simulink library "LibraryExperimental"  (R2013b)
settings: Solver=ode45  StartTime=0.0  StopTime=10.0  RelTol=1e-3
values from neighbouring files (symbols this model uses):
  dimActuator = 24    [init_experimental_setup.m]
  layoutActuator = actuatorPlace    [init_experimental_setup.m]
undefined symbols (not defined in the file or in its folder): ident_normalized_static, ultidyn
undefined symbols (not defined in the file): delayWavefrontEthernet, dimSlopeMatrix, dimSquareMatrix, DMmodel, DMmodel_static, sampleTimeTipTilt, sampleTimeWavefrontSensor, staticDMInput, strokeTipTiltMirror
libraries: RCTblocks x1
settings Model: Creator=smauch  LastModifiedBy=smauch

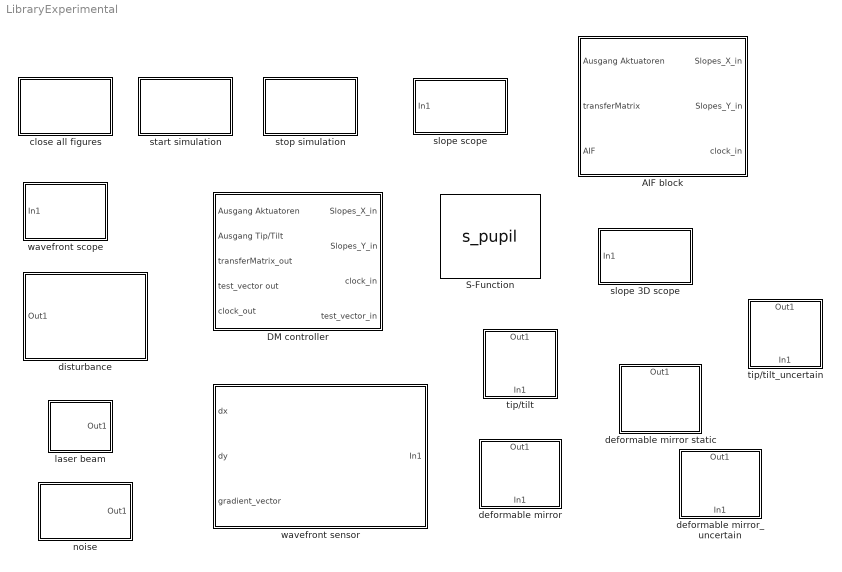
== system LibraryExperimental ==
  AIF block : Subsystem  mask{nbAct=24}
      mask prompts: nbAct "number of actuators"
      mask Display:
      | image(imread('controller.jpg'))
      | color('blue');
      | patch( [0 0.3 0.3 0], [0.9 0.9 0.75 0.75], [0.9, 0.9, 0.9] )
      | port_label('output', 1, 'y')
      | patch( [0 0.5 0.5 0], [0.425 0.425 0.575 0.575], [0.9, 0.9, 0.9] )
      | port_label('output', 2, 'actuator_matrix')
      | patch( [0 0.5 0.5 0], [0.1 0.1 0.25 0.25], [0.9, 0.9, 0.9] )
      | port_label('output', 3, 'AIF_matrix')
      | 
      | patch( [1 0.875 0.875 1], [0.9 0.9 0.75 0.75], [0.9, 0.9, 0.9] )
      | port_label('input', 1, 'dx')
      | patch( [1 0.875 0.875 1], [0.45 0.45 0.55 0.55], [0.9, 0.9, 0.9] )
      | port_label('input', 2, 'dy')
      | patch( [1 0.8 0.8 1], [0.1 0.1 0.25 0.25], [0.9, 0.9, 0.9] )
      | port_label('input', 3, 'clock')
  DM controller : Subsystem
      mask Display:
      | image(imread('controller.jpg'))
      | color('blue');
      | port_label('output', 1, 'y')
      | port_label('output', 2, 'tip/tilt')
      | port_label('output', 3, 'actuator_matrix')
      | 
      | port_label('input', 1, 'dx')
      | port_label('input', 2, 'dy')
      | port_label('input', 3, 'clock')
  S-Function : S-Function  FunctionName=s_pupil  Parameters=dimMatrix  EnableBusSupport=off  mask{dimMatrix=dimSquareMatrix}
      mask prompts: dimMatrix "dimension of input/outut matrix"
      mask Display:
      | t = 0:0.1:2*pi;
      | x = (cos(t)+1)/2;
      | y = (sin(t)+1)/2;
      | patch(x,y,[0 0 0])
      | color('white')
      | fprintf('round\npupil')
  close all figures : Subsystem
      settings: OpenFcn=close all;
      mask Display:
      | patch([0 0 1 1], [0 20 20 0],[1 0 0])
      | color('black')
      | fprintf('close all\nfigures')
  deformable mirror : Subsystem  mask{dimActuator=dimActuator, dimMatrix=dimSquareMatrix, layoutActuator=layoutActuator, model=DMmodel}
      mask prompts: dimActuator "# Actuator"; dimMatrix "dimSquareMatrix"; layoutActuator "layout actuator to dimSquareMatrix"; model "state space model"
      mask Display:
      | image(imread('dm.jpg'))
      | color('white');
      | 
      | port_label('output', 1, 'y')
      | port_label('input', 1, 'u')
      | 
      | patch( [0.15 0.85 0.85 0.15], [0.2 0.2 0.8 0.8], [0 0 0])
      | color('white');
      | fprintf('level 2\ns-function\nuncertain')
  deformable mirror static : Subsystem  mask{dimActuator=dimActuator, dimMatrix=dimSquareMatrix, layoutActuator=layoutActuator, dm_static=DMmodel_static, input=staticDMInput, delay=1}
      mask prompts: dimActuator "# Actuator"; dimMatrix "dimSquareMatrix"; layoutActuator "layout actuator to dimSquareMatrix"; dm_static "static DM model"; input "input for static DM"; delay "delay of disturbance in seconds"
      mask Display:
      | image(imread('dm.jpg'))
      | color('white');
      | 
      | port_label('output', 1, 'y')
      | 
      | patch( [0.15 0.85 0.85 0.15], [0.2 0.2 0.8 0.8], [0 0 0])
      | color('white');
      | fprintf('level 2\ns-function\nstatic')
  deformable mirror_uncertain : Subsystem  AncestorBlock=LibraryExperimental/deformable mirror  mask{Parameter6=0, dimMatrix=dimSquareMatrix, layoutActuator=layoutActuator, model=DMmodel, uncertainty=1/5, ident_normalized_static=ident_normalized_static}
      mask prompts: dimMatrix "dimSquareMatrix"; layoutActuator "layout actuator to dimSquareMatrix"; model "state space model"; uncertainty "uncertainty (normalized)"
      mask Display:
      | image(imread('dm.jpg'))
      | color('white');
      | 
      | port_label('output', 1, 'y')
      | port_label('input', 1, 'u')
      | 
      | patch( [0.15 0.85 0.85 0.15], [0.2 0.2 0.8 0.8], [0 0 0])
      | color('white');
      | fprintf('level 2\ns-function\nuncertain')
  disturbance : Subsystem  mask{dimMatrix=dimSquareMatrix, zernik1=1, zernik2=-1, scale=5, rotate=45}
      mask prompts: dimMatrix "dimSquareMatrix"; zernik1 "Zernike1"; zernik2 "Zernike2"; rotate "rotate in deg"
      mask Display:
      | port_label('output', 1, 'y')
      | 
      | patch([0 0.5 1], [0 1 0],[0.7 0.6 0])
      | patch( [0.15 0.85 0.85 0.15], [0.6 0.6 0.4 0.4], [0.9 0.9 0.9] )
      | fprintf('stationar Zernike')
  laser beam : Subsystem  mask{dimSquare=dimSquareMatrix}
      mask prompts: dimSquare "dimSquareMatrix"
      mask Display:
      | %patch([0 0.5 1], [0 1 0],[0.9 0.3 0.5])
      | image('laser.jpg')
      | patch( [0 1 1 0], [0.8 0.8 0.45 0.45], [0.9 0.9 0.9] )
      | fprintf('laser beam\n')
  noise : Subsystem  mask{enable=on, dimSquare=dimSquareMatrix, Ts=-1, scaleNoise=1}
      mask prompts: enable "enable noise"; dimSquare "dimSquareMatrix"; Ts "sample time"; scaleNoise "noise scaling (default is rand)"
      mask Display:
      | patch([0 0.5 1], [0 1 0],[0.9 0.3 0.5])
      | patch( [0.15 0.85 0.85 0.15], [0.75 0.75 0.25 0.25], [0.9 0.9 0.9] )
      | fprintf('noise\ngeneration')
  slope 3D scope : Subsystem  mask{sampleTime=0.1, dimMatrix=dimSlopeMatrix, enable=on, title='3D wavefront sensor'}
      mask prompts: sampleTime "Sample Time"; dimMatrix "dimSquareMatrix"; enable "enable Scope"
      mask Display:
      | patch([0 0.5 1], [0 1 0],[1 0 0])
      | patch( [0.15 0.85 0.85 0.15], [0.6 0.6 0.4 0.4], [0.9 0.9 0.9] )
      | fprintf('Scope 3D SHWFS')
  slope scope : Subsystem  mask{sampleTime=0.1, dimMatrix=dimSlopeMatrix, enable=on, title='wavefront sensor'}
      mask prompts: sampleTime "Sample Time"; dimMatrix "dimSquareMatrix"; enable "enable Scope"
      mask Display:
      | patch([0 0.5 1], [0 1 0],[1 0 0])
      | patch( [0.15 0.85 0.85 0.15], [0.6 0.6 0.4 0.4], [0.9 0.9 0.9] )
      | fprintf('Scope Quiver')
  start simulation : Subsystem
      settings: OpenFcn=set_param(gcs, 'SimulationCommand', 'start')
      mask Display:
      | patch([0 0 1 1], [0 20 20 0],[0 1 0])
      | color('black')
      | fprintf('start\nsimulation')
  stop simulation : Subsystem
      settings: OpenFcn=set_param(gcs, 'SimulationCommand', 'stop')
      mask Display:
      | patch([0 0 1 1], [0 20 20 0],[1 0 0])
      | color('black')
      | fprintf('stop\nsimulation')
  tip/tilt : Subsystem  mask{sampleTime=sampleTimeTipTilt, dimMatrix=dimSquareMatrix, strokeTipTilt=strokeTipTiltMirror, enableDyn=on, enableLimit=on}
      mask prompts: sampleTime "Sample Time"; dimMatrix "dimSquareMatrix"; strokeTipTilt "stroke tip-tilt mirror"; enableDyn "enableDynamic"; enableLimit "enableLimiter"
      mask Display:
      | image(imread('dm.jpg'))
      | color('white');
      | 
      | port_label('output', 1, 'y')
      | port_label('input', 1, 'u')
      | 
      | patch( [0.15 0.85 0.85 0.15], [0.4 0.4 0.6 0.6], [0 0 0])
      | color('white');
      | fprintf('uncertain')
  tip/tilt_uncertain : Subsystem  AncestorBlock=LibraryExperimental/tip//tilt  mask{sampleTime=sampleTimeTipTilt, dimMatrix=dimSquareMatrix, strokeTipTilt=strokeTipTiltMirror, enableDyn=on, enableLimit=on}
      mask prompts: sampleTime "Sample Time"; dimMatrix "dimSquareMatrix"; strokeTipTilt "stroke tip-tilt mirror"; enableDyn "enableDynamic"; enableLimit "enableLimiter"
      mask Display:
      | image(imread('dm.jpg'))
      | color('white');
      | 
      | port_label('output', 1, 'y')
      | port_label('input', 1, 'u')
      | 
      | patch( [0.15 0.85 0.85 0.15], [0.4 0.4 0.6 0.6], [0 0 0])
      | color('white');
      | fprintf('uncertain')
  wavefront scope : Subsystem  mask{sampleTime=0.1, dimMatrix=dimSquareMatrix, enable=on, title='disturbance'}
      mask prompts: sampleTime "Sample Time"; dimMatrix "dimSquareMatrix"; enable "enable Scope"
      mask Display:
      | patch([0 0.5 1], [0 1 0],[1 0 0])
      | patch( [0.15 0.85 0.85 0.15], [0.6 0.6 0.4 0.4], [0.9 0.9 0.9] )
      | fprintf('Scope surf')
  wavefront sensor : Subsystem  mask{sampleTime=sampleTimeWavefrontSensor, dimMatrix_i=dimSquareMatrix, dimMatrix_o=dimSlopeMatrix, delay=delayWavefrontEthernet, noiseSHWFS=0, scaleSHWFS=1, aperture=on}
      mask prompts: sampleTime "sample time of SHWFS"; dimMatrix_i "dimSquareMatrix Input"; dimMatrix_o "dimSquareMatrix Output"; delay "delay of SHWFS in ms"; noiseSHWFS "SHWFS noise"; scaleSHWFS "SHWFS scale"; aperture "enable circular aperture"
      mask Display:
      | image(imread('shacksensor.jpg'))
      | 
      | patch( [1 1 0.9 0.9],[0.4 0.6 0.6 0.4],[0.9 0.9 0.9] )
      | port_label('input', 1, 'u')
      | 
      | patch( [0 0 0.1 0.1],[0.9 0.75 0.75 0.9],[0.9 0.9 0.9] )
      | port_label('output', 1, 'dx')
      | 
      | patch( [0 0 0.1 0.1],[0.425 0.575 0.575 0.425],[0.9 0.9 0.9] )
      | port_label('output', 2, 'dy')
      | 
      | patch( [0 0 0.25 0.25],[0.1 0.25 0.25 0.1],[0.9 0.9 0.9] )
      | port_label('output', 3, 'wavefront')

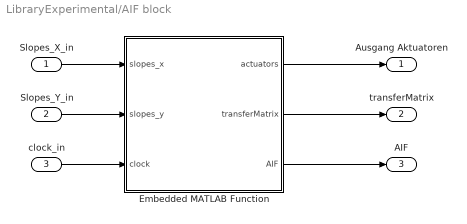
== system LibraryExperimental/AIF block ==
  Slopes_X_in : Inport
  Slopes_Y_in : Inport  Port=2
  clock_in : Inport  Port=3
  Embedded MATLAB Function : MATLAB Function  TreatAsAtomicUnit=on
  Ausgang Aktuatoren : Outport
  transferMatrix : Outport  Port=2
  AIF : Outport  Port=3
  wires:
  Slopes_X_in/1 -> Embedded MATLAB Function/1(slopes_x)
  Slopes_Y_in/1 -> Embedded MATLAB Function/2(slopes_y)
  clock_in/1 -> Embedded MATLAB Function/3(clock)
  Embedded MATLAB Function/2(transferMatrix) -> transferMatrix/1
  Embedded MATLAB Function/3(AIF) -> AIF/1
  Embedded MATLAB Function/1(actuators) -> Ausgang Aktuatoren/1

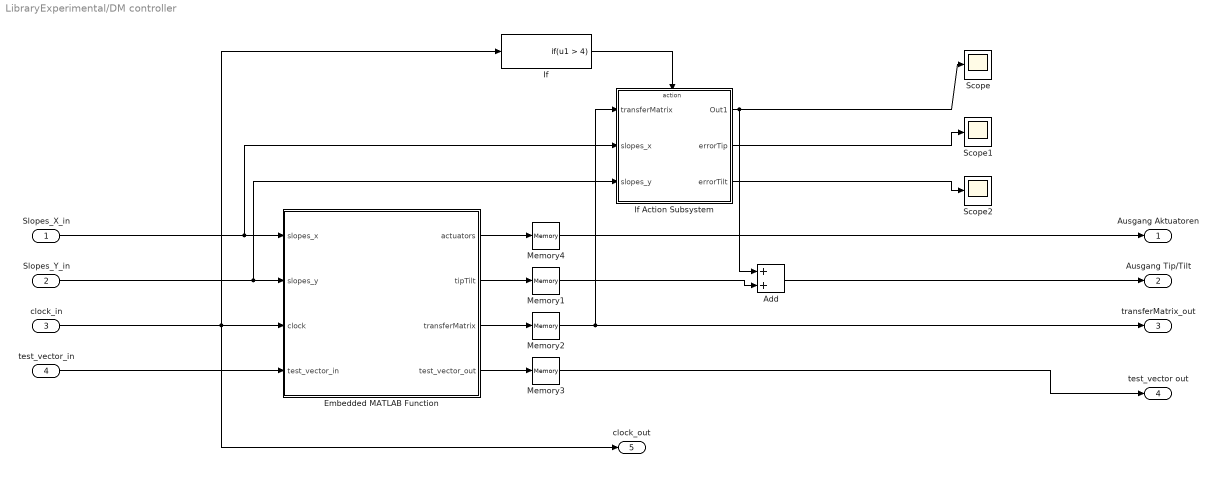
== system LibraryExperimental/DM controller ==
  Slopes_X_in : Inport
  Slopes_Y_in : Inport  Port=2
  clock_in : Inport  Port=3
  test_vector_in : Inport  Port=4
  Add : Sum
  Embedded MATLAB Function : MATLAB Function  TreatAsAtomicUnit=on
  If : If  IfExpression=u1 > 4  ShowElse=off
  If Action Subsystem : Subsystem  TreatAsAtomicUnit=on
  Memory{1..4} (4 alike) : Memory  InheritSampleTime=on
  Scope : Scope
      settings: YMin=-0.65  YMax=0.05
  Scope1 : Scope
      settings: TimeRange=0.07317073170731714  YMin=-0.00055  YMax=0.0004
  Scope2 : Scope
      settings: TimeRange=0.07317073170731714  YMin=-1.4  YMax=0.7  SaveName=ScopeData2
  Ausgang Aktuatoren : Outport
  Ausgang Tip/Tilt : Outport  Port=2
  transferMatrix_out : Outport  Port=3
  test_vector out : Outport  Port=4
  clock_out : Outport  Port=5
  wires:
  Memory3/1 -> test_vector out/1
  If Action Subsystem/3(errorTilt) -> Scope2/1
  If Action Subsystem/2(errorTip) -> Scope1/1
  If Action Subsystem/1(Out1) -> Scope/1, Add/1
  If/1 -> If Action Subsystem/Action
  Add/1 -> Ausgang Tip/Tilt/1
  Memory1/1 -> Add/2
  Embedded MATLAB Function/3(transferMatrix) -> Memory2/1
  Memory2/1 -> If Action Subsystem/1(transferMatrix), transferMatrix_out/1
  Memory4/1 -> Ausgang Aktuatoren/1
  test_vector_in/1 -> Embedded MATLAB Function/4(test_vector_in)
  clock_in/1 -> Embedded MATLAB Function/3(clock), If/1, clock_out/1
  Slopes_Y_in/1 -> Embedded MATLAB Function/2(slopes_y), If Action Subsystem/3(slopes_y)
  Slopes_X_in/1 -> Embedded MATLAB Function/1(slopes_x), If Action Subsystem/2(slopes_x)
  Embedded MATLAB Function/4(test_vector_out) -> Memory3/1
  Embedded MATLAB Function/2(tipTilt) -> Memory1/1
  Embedded MATLAB Function/1(actuators) -> Memory4/1

== system LibraryExperimental/close all figures ==

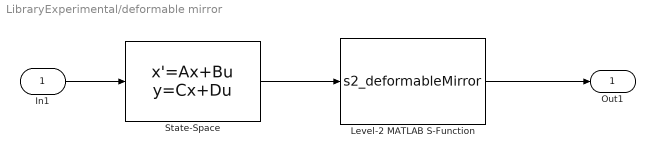
== system LibraryExperimental/deformable mirror ==
  In1 : Inport
  Level-2 MATLAB S-Function : M-S-Function  FunctionName=s2_deformableMirror  Parameters=dimActuator,dimMatrix,layoutActuator
  State-Space : StateSpace  A=model.A  B=model.B  C=model.C  D=model.D  X0=0
  Out1 : Outport
  wires:
  Level-2 MATLAB S-Function/1 -> Out1/1
  In1/1 -> State-Space/1
  State-Space/1 -> Level-2 MATLAB S-Function/1

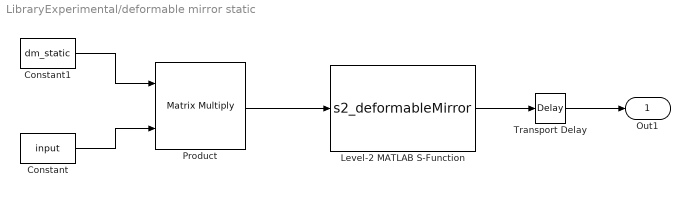
== system LibraryExperimental/deformable mirror static ==
  Constant : Constant  Value=input  VectorParams1D=off
  Constant1 : Constant  Value=dm_static
  Level-2 MATLAB S-Function : M-S-Function  FunctionName=s2_deformableMirror  Parameters=dimActuator,dimMatrix,layoutActuator
  Product : Product  Multiplication=Matrix(*)
  Transport Delay : TransportDelay  DelayTime=delay  PadeOrder=3
  Out1 : Outport
  wires:
  Level-2 MATLAB S-Function/1 -> Transport Delay/1
  Product/1 -> Level-2 MATLAB S-Function/1
  Constant1/1 -> Product/1
  Constant/1 -> Product/2
  Transport Delay/1 -> Out1/1

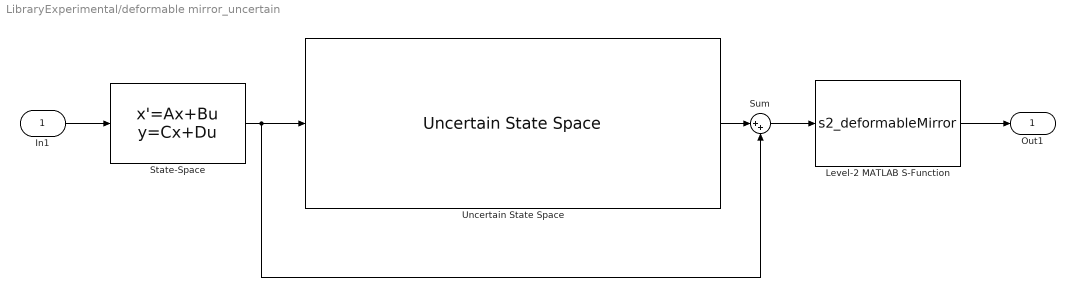
== system LibraryExperimental/deformable mirror_uncertain ==
  In1 : Inport
  Level-2 MATLAB S-Function : M-S-Function  FunctionName=s2_deformableMirror  Parameters=dimActuator,dimMatrix,layoutActuator
  State-Space : StateSpace  A=model.A  B=model.B  C=model.C  D=model.D  X0=0
  Sum : Sum  Inputs=|++
  Uncertain State Space : RCTblocks/Uncertain State Space  Tag=USS  USystem=ident_normalized_static*ultidyn( 'deltaDM',[dimActuator dimActuator],'Bound',1)*uncertainty  UValue=uval  X0=[]  uX0=[]
  Out1 : Outport
  wires:
  In1/1 -> State-Space/1
  Level-2 MATLAB S-Function/1 -> Out1/1
  Sum/1 -> Level-2 MATLAB S-Function/1
  State-Space/1 -> Sum/2, Uncertain State Space/1
  Uncertain State Space/1 -> Sum/1

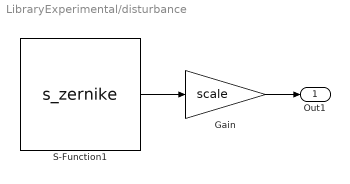
== system LibraryExperimental/disturbance ==
  Gain : Gain  Gain=scale
  S-Function1 : S-Function  FunctionName=s_zernike  Parameters=dimMatrix,zernik1,zernik2,rotate  EnableBusSupport=off
  Out1 : Outport
  wires:
  S-Function1/1 -> Gain/1
  Gain/1 -> Out1/1

== system LibraryExperimental/laser beam ==
  laser beam : Constant  Value=zeros(dimSquare.^2,1)
  Out1 : Outport
  wires:
  laser beam/1 -> Out1/1

== system LibraryExperimental/noise ==
  white noise disturbances : MATLABFcn  MATLABFcn=rand(dimSquare.^2,1)*enable*scaleNoise  SampleTime=Ts
  Out1 : Outport
  wires:
  white noise disturbances/1 -> Out1/1

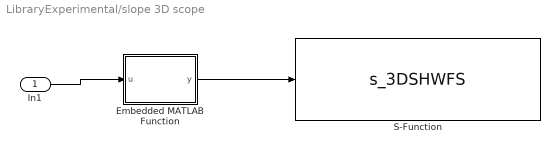
== system LibraryExperimental/slope 3D scope ==
  In1 : Inport
  Embedded MATLAB Function : MATLAB Function  TreatAsAtomicUnit=on
  S-Function : S-Function  FunctionName=s_3DSHWFS  Parameters=sampleTime,dimMatrix,enable,title  EnableBusSupport=off
  wires:
  In1/1 -> Embedded MATLAB Function/1(u)
  Embedded MATLAB Function/1(y) -> S-Function/1

== system LibraryExperimental/slope scope ==
  In1 : Inport
  Embedded MATLAB Function : MATLAB Function  TreatAsAtomicUnit=on
  S-Function : S-Function  FunctionName=s_quiver  Parameters=sampleTime,dimMatrix,enable,title  EnableBusSupport=off
  wires:
  In1/1 -> Embedded MATLAB Function/1(u)
  Embedded MATLAB Function/1(y) -> S-Function/1

== system LibraryExperimental/start simulation ==

== system LibraryExperimental/stop simulation ==

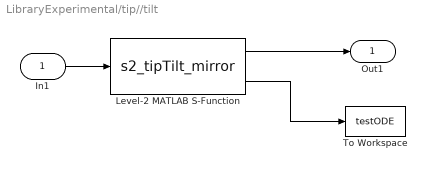
== system LibraryExperimental/tip//tilt ==
  In1 : Inport
  Level-2 MATLAB S-Function : M-S-Function  FunctionName=s2_tipTilt_mirror  Parameters=sampleTime,dimMatrix,strokeTipTilt,enableDyn,enableLimit
  To Workspace : ToWorkspace  VariableName=testODE  SampleTime=-1  SaveFormat=Structure
  Out1 : Outport
  wires:
  Level-2 MATLAB S-Function/2 -> To Workspace/1
  In1/1 -> Level-2 MATLAB S-Function/1
  Level-2 MATLAB S-Function/1 -> Out1/1

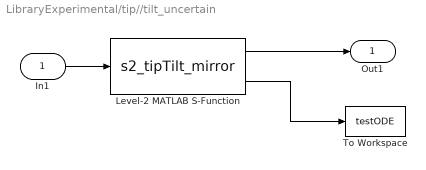
== system LibraryExperimental/tip//tilt_uncertain ==
  In1 : Inport
  Level-2 MATLAB S-Function : M-S-Function  FunctionName=s2_tipTilt_mirror  Parameters=sampleTime,dimMatrix,strokeTipTilt,enableDyn,enableLimit
  To Workspace : ToWorkspace  VariableName=testODE  SampleTime=-1  SaveFormat=Structure
  Out1 : Outport
  wires:
  Level-2 MATLAB S-Function/1 -> Out1/1
  In1/1 -> Level-2 MATLAB S-Function/1
  Level-2 MATLAB S-Function/2 -> To Workspace/1

== system LibraryExperimental/wavefront scope ==
  In1 : Inport
  Embedded MATLAB Function : MATLAB Function  TreatAsAtomicUnit=on
  S-Function : S-Function  FunctionName=s_surf  Parameters=sampleTime,dimMatrix,enable,title  EnableBusSupport=off
  wires:
  In1/1 -> Embedded MATLAB Function/1(u)
  Embedded MATLAB Function/1(y) -> S-Function/1

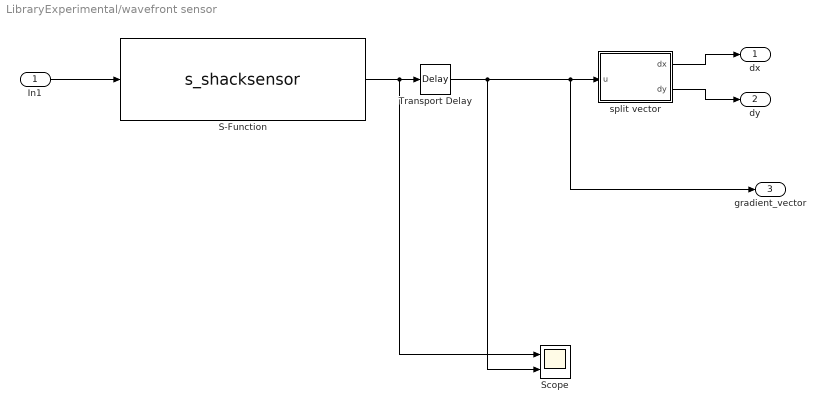
== system LibraryExperimental/wavefront sensor ==
  In1 : Inport
  S-Function : S-Function  FunctionName=s_shacksensor  Parameters=sampleTime,dimMatrix_i,dimMatrix_o,noiseSHWFS,scaleSHWFS,aperture  EnableBusSupport=off
  Scope : Scope  NumInputPorts=2
      settings: YMin=-5~-5  YMax=5~5  SaveName=ScopeData3
  Transport Delay : TransportDelay  DelayTime=delay*10^(-3)
  split vector : MATLAB Function  TreatAsAtomicUnit=on
  dx : Outport
  dy : Outport  Port=2
  gradient_vector : Outport  Port=3
  wires:
  split vector/1(dx) -> dx/1
  split vector/2(dy) -> dy/1
  In1/1 -> S-Function/1
  S-Function/1 -> Scope/1, Transport Delay/1
  Transport Delay/1 -> Scope/2, gradient_vector/1, split vector/1(u)

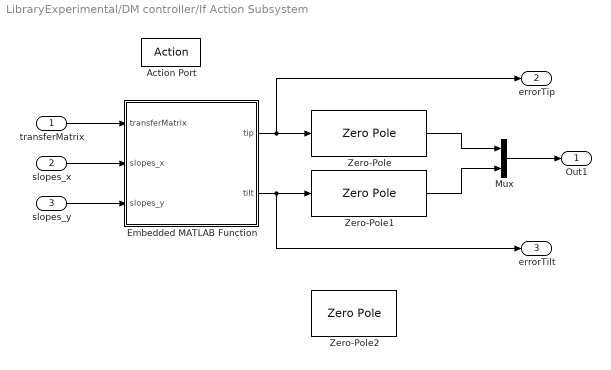
== system LibraryExperimental/DM controller/If Action Subsystem ==
  transferMatrix : Inport
  slopes_x : Inport  Port=2
  slopes_y : Inport  Port=3
  Action Port : ActionPort
  Embedded MATLAB Function : MATLAB Function  TreatAsAtomicUnit=on
  Mux : Mux  Inputs=2
  Zero-Pole : ZeroPole  Zeros=[-2800]  Poles=[0]  Gain=[-100/2800]
  Zero-Pole1 : ZeroPole  Zeros=[-2800]  Poles=[0]  Gain=[-100/2800]
  Zero-Pole2 : ZeroPole  Zeros=[-450]  Poles=[0]  Gain=[-80/450]
  Out1 : Outport
  errorTip : Outport  Port=2
  errorTilt : Outport  Port=3
  wires:
  Zero-Pole1/1 -> Mux/2
  Zero-Pole/1 -> Mux/1
  Embedded MATLAB Function/2(tilt) -> Zero-Pole1/1, errorTilt/1
  Embedded MATLAB Function/1(tip) -> errorTip/1, Zero-Pole/1
  slopes_y/1 -> Embedded MATLAB Function/3(slopes_y)
  slopes_x/1 -> Embedded MATLAB Function/2(slopes_x)
  transferMatrix/1 -> Embedded MATLAB Function/1(transferMatrix)
  Mux/1 -> Out1/1

== matlab function LibraryExperimental/AIF block/Embedded MATLAB Function ==
  data: slopes_x input size=[196]; slopes_y input size=[196]; nbAct parameter; actuators output; clock input; transferMatrix output; AIF output
function [actuators, transferMatrix, AIF] = fcn(slopes_x, slopes_y, nbAct, clock)
% this embedded MATLAB block creates the transfer matrix
% by simply actuating every actuator and using the resulting slopes
% to get the transfer matrix
%
% (c) 2011-215 Steffen Mauch, Ingenieurbuero Mauch - Unorthodox Solutions
%

persistent actuatorfunction;
persistent actuators_old;
persistent k;
persistent slope_zero_x;
persistent slope_zero_y;
persistent old_clock;
persistent transferMatrix_old;

sizeSlopes = size(slopes_x,1);

if isempty(actuatorfunction)
   actuatorfunction = zeros( sizeSlopes*2, nbAct ); 
end

%#coder   
coder.extrinsic('actuators', 'linspace');

if isempty(actuators_old)
   actuators_old = zeros(nbAct,1); 
end

if isempty(k)
   k = 0; 
end

if isempty(old_clock)
   old_clock = 0; 
end

if isempty(transferMatrix_old)
   transferMatrix_old = zeros( nbAct, sizeSlopes*2 );
end

if isempty(slope_zero_x)
   slope_zero_x = zeros( sizeSlopes, 1 ); 
end
if isempty(slope_zero_y)
   slope_zero_y = zeros( sizeSlopes, 1 ); 
end

actuators       = actuators_old;  %auf letzte ausgegebene werte setzen (bei letztem clockwechsel..)
transferMatrix  = transferMatrix_old;

% [k] is 1/100 seconds
if( floor(old_clock*100) < floor(clock*100) )
    k = k + 1;
        
    % hier wird die Akturatoreinflussfunktion aufgenommen
    if( k == 1 )
        slope_zero_x = slopes_x;
        slope_zero_y = slopes_y;
    end
    for m = 1:nbAct
        if( (k >= m*20-15) && (k <= m*20+14) )
           actuators(:) = 0;
           actuators(m) = 1; 
        end
        if( k >= m*20-2 && k <= m*20+2 )
            actuatorfunction(:,m) = [(slopes_x - slope_zero_x); (slopes_y - slope_zero_y)] ;
        end
    end
    
    if( k >= nbAct*20+10 && k <= nbAct*20+15 )
        transferMatrix = inv(actuatorfunction.'*actuatorfunction)*actuatorfunction.';
    end
    
    actuators_old = actuators;            %save values until..clock change
    transferMatrix_old  = transferMatrix;

end

AIF             = actuatorfunction;
old_clock       = clock;

== matlab function LibraryExperimental/slope 3D scope/Embedded MATLAB Function ==
  data: u input; y output
function y = fcn(u)
%#eml

y = u(:);

== matlab function LibraryExperimental/slope scope/Embedded MATLAB Function ==
  data: u input; y output
function y = fcn(u)
%#eml

y = u(:);

== matlab function LibraryExperimental/DM controller/If Action Subsystem/Embedded MATLAB Function ==
  data: transferMatrix input; slopes_x input size=[196]; slopes_y input size=[196]; tip output; tilt output
function [tip, tilt] = fcn(transferMatrix, slopes_x, slopes_y)

 a=transferMatrix*[slopes_x; slopes_y];
 tip = a(1);
 tilt = a(2);

== matlab function LibraryExperimental/DM controller/Embedded MATLAB Function ==
  data: slopes_x input size=[196]; slopes_y input size=[196]; actuators output; clock input; tipTilt output; transferMatrix output size=[2 392]; test_vector_in input; test_vector_out output
function [actuators,tipTilt,transferMatrix, test_vector_out] = fcn(slopes_x, slopes_y, clock, test_vector_in)
% this embedded MATLAB block creates the transfer matrix
% by simply actuating every actuator and using the resulting slopes
% to get the transfer matrix
%
% (c) 04/2011 Steffen Mauch, TU Ilmenau
% Version: 0.02 alpha
%
% usage for example with MATLAB
%   sim('erzeugungDerMatrix',[0 16],[],[creataData(16)])
%
% changelog:
%  - initial design (date: 2011-04-04, 0.01 alpha)
%  - changed input to slope_x and slope_y (date: 2011-04-05, 0.02 alpha)

persistent actuatorfunction;
persistent actuators_old;
persistent tipTilt_old;
persistent k;
persistent slope_zero_x;
persistent slope_zero_y;
persistent old_clock;
persistent transferMatrix_inside;
persistent transferMatrix_old;

%persistent transferMatrix; %persistent nicht für outputs..


if isempty(actuatorfunction)
   %actuatorfunction = zeros(size(slopes_x,1)*2,13); 
   actuatorfunction = zeros(size(slopes_x,1)*2,2); 
end

if isempty(actuators_old)
   actuators_old = zeros(1,13); 
end

if isempty(tipTilt_old)
   tipTilt_old = [0 0]; 
end

if isempty(k)
   k = 0; 
end

if isempty(old_clock)
   old_clock = 0; 
end

if isempty(transferMatrix_inside)
   %transferMatrix_inside = zeros(13,196*2);
   transferMatrix_inside = zeros(2,196*2);
end

if isempty(transferMatrix_old)
   %transferMatrix_old = zeros(13,196*2);
   transferMatrix_old = zeros(2,196*2);
end

if isempty(slope_zero_x)
   slope_zero_x = zeros(196,1); 
end
if isempty(slope_zero_y)
   slope_zero_y = zeros(196,1); 
end

actuators = actuators_old;  %auf letzte ausgegebene werte setzen (bei letztem clockwechsel..)
tipTilt = tipTilt_old;
transferMatrix = transferMatrix_old; %auf letzte ausgegebene werte setzen (bei letztem clockwechsel..)
clock_change = false;

% if( floor(old_clock) < floor(clock) )
%     k = k+1;
%         
%     % hier wird die Akturatoreinflussfunktion aufgenommen
%     if( k >= 1 && k <= 13)
%         tipTilt = [0.5 1];
%         if k == 1
%             slope_zero_x = slopes_x;
%             slope_zero_y = slopes_y;
%         else
%             actuatorfunction(:,k-1) = [(slopes_x - slope_zero_x); (slopes_y - slope_zero_y)] ;
%         end
%         actuators = zeros(1,13);
%         actuators(k)=200;
%     elseif( k == 14 )
%         actuatorfunction(:,13) = [(slopes_x - slope_zero_x); (slopes_y - slope_zero_y)];
%     elseif(k == 15 )
%         %size(actuatorfunction);
%         
%         transferMatrix = inv(actuatorfunction.'*actuatorfunction)*actuatorfunction.';
%     end
%     
%     actuators_old=actuators;            %save values until..clock change
%     transferMatrix_old=transferMatrix;  %save values until..clock change
% end




%% TIP-TILT
% change 13.01.2012 (c) Steffen Mauch
% [k] is now 1/10 seconds, not seconds anymore
if( floor(old_clock*10) < floor(clock*10) )
    k = k+1;
        
    % hier wird die Akturatoreinflussfunktion aufgenommen
    if( k < 40)
        if k == 4
            slope_zero_x = slopes_x;
            slope_zero_y = slopes_y;
        elseif( k >= 5 && k < 10 )
            tipTilt=[(k-4)/5 0];
        elseif( k == 14 )
            actuatorfunction(:,1) = [(slopes_x - slope_zero_x); (slopes_y - slope_zero_y)] ;
        elseif( k >= 15 && k < 20 )
            tipTilt=[1-(k-14)/5 0];
        elseif( k >= 25 && k < 30 )
            tipTilt=[0 (k-24)/5];
        elseif( k == 34 )
            actuatorfunction(:,2) = [(slopes_x - slope_zero_x); (slopes_y - slope_zero_y)] ;
        elseif( k >= 35 && k<40 )
            tipTilt=[0 1-(k-34)/5];
        end
    elseif(k == 40 )
        transferMatrix = inv(actuatorfunction.'*actuatorfunction)*actuatorfunction.';
    end
    
    actuators_old=actuators;            %save values until..clock change
    transferMatrix_old=transferMatrix;  %save values until..clock change
    
    % ab hier wird dann geregelt!
    if(  k > 40 )
        ;
    end  
end




 

old_clock = clock;
tipTilt_old = tipTilt;
test_vector_out=test_vector_in;
test_vector_out(1)=clock;

== matlab function LibraryExperimental/wavefront sensor/split vector ==
  data: dx output; u input; dy output
function [dx,dy] = fcn(u)
%#eml
u_length = length(u);

dx = u(1:u_length/2);
dy = u(u_length/2+1:u_length);

== matlab function LibraryExperimental/wavefront scope/Embedded MATLAB Function ==
  data: u input; y output
function y = fcn(u)
%#eml

y = u(:);
